simulink model "System"  (R2020b)
settings: Solver=VariableStepAuto  StartTime=0.0  StopTime=100  MaxStep=0.001  RelTol=1e-3
PreLoadFcn:
  | M1 = 1200;
  | k1 = 21000;
  | b = 2500;
  | M2 = 13;
  | k2 = 320;
settings Model: Creator=smart  LastModifiedBy=smart

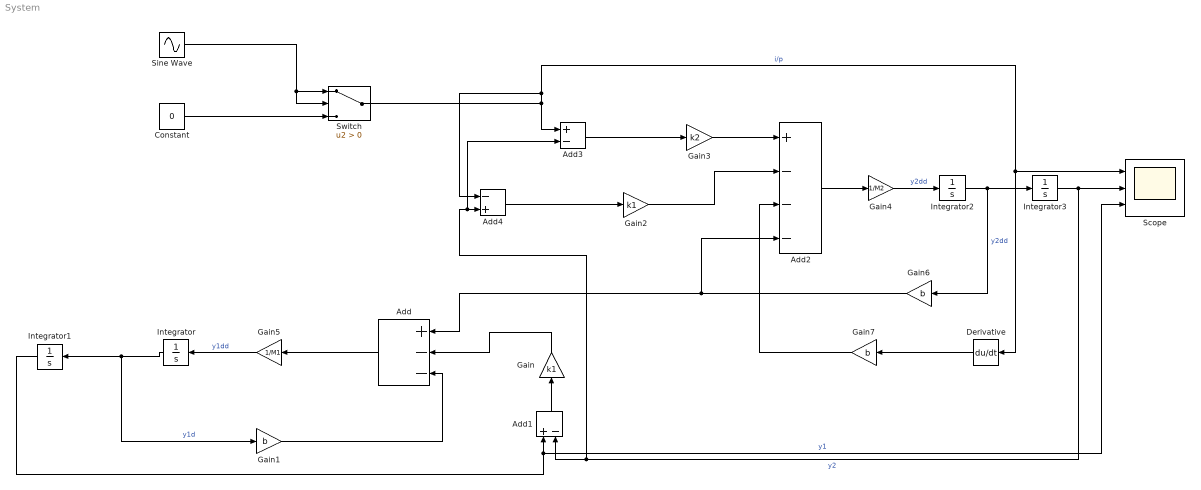
== system System ==
  Add : Sum  Inputs=+--
  Add1 : Sum  Inputs=+-
  Add2 : Sum  Inputs=+---
  Add3 : Sum  Inputs=+-
  Add4 : Sum  Inputs=-+
  Constant : Constant  Value=0
  Derivative : Derivative
  Gain : Gain  Gain=k1
  Gain1 : Gain  Gain=b
  Gain2 : Gain  Gain=k1
  Gain3 : Gain  Gain=k2
  Gain4 : Gain  Gain=1/M2
  Gain5 : Gain  Gain=1/M1
  Gain6 : Gain  Gain=b
  Gain7 : Gain  Gain=b
  Integrator{,1..3} (4 alike) : Integrator
  Scope : Scope  NumInputPorts=3
  Sine Wave : Sin  Frequency=0.1  SampleTime=0
  Switch : Switch  Criteria=u2 > Threshold
  wires:
  Gain1/1 -> Add/3
  Add/1 -> Gain5/1
  Gain5/1 -> Integrator/1  "y1dd"
  Integrator/1 -> Gain1/1, Integrator1/1  "y1d"
  Gain/1 -> Add/2
  Add1/1 -> Gain/1
  Integrator1/1 -> Scope/3, Add1/1  "y1"
  Gain3/1 -> Add2/1
  Gain2/1 -> Add2/2
  Add4/1 -> Gain2/1
  Add3/1 -> Gain3/1
  Integrator3/1 -> Scope/2, Add3/2, Add4/2, Add1/2  "y2"
  Add2/1 -> Gain4/1
  Gain4/1 -> Integrator2/1  "y2dd"
  Integrator2/1 -> Gain6/1, Integrator3/1  "y2dd"
  Gain6/1 -> Add2/4, Add/1
  Gain7/1 -> Add2/3
  Derivative/1 -> Gain7/1
  Switch/1 -> Scope/1, Derivative/1, Add4/1, Add3/1  "i/p"
  Sine Wave/1 -> Switch/2, Switch/1
  Constant/1 -> Switch/3
